simulink model "model"  (Simulink 7.8)
settings: Solver=ode45  StartTime=0.0  StopTime=40.0  RelTol=1e-3
libraries: simulink x2
settings Model: Creator=nort  LastModifiedBy=nort

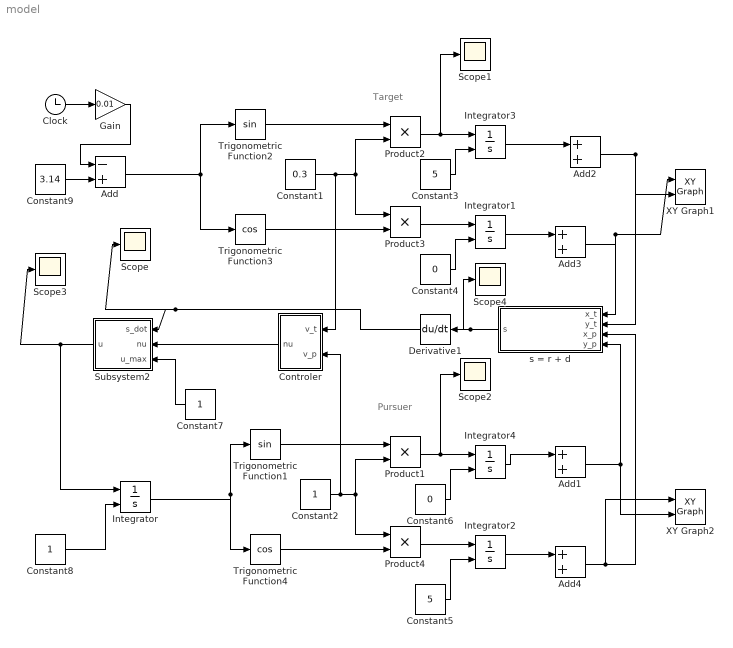
== system model ==
  note: Target
  note: Pursuer
  Add : Sum  Inputs=-+
  Add{1..4} (4 alike) : Sum
  Clock : Clock
  Constant1 : Constant  Value=0.3
  Constant2 : Constant
  Constant3 : Constant  Value=5
  Constant4 : Constant  Value=0
  Constant5 : Constant  Value=5
  Constant6 : Constant  Value=0
  Constant7 : Constant
  Constant8 : Constant
  Constant9 : Constant  Value=3.14
  Controler : Subsystem
  Derivative1 : Derivative
  Gain : Gain  Gain=0.01
  Integrator : Integrator  InitialConditionSource=external  InitialCondition=3.14/4
  Integrator{1..4} (4 alike) : Integrator  InitialConditionSource=external
  Product{1..4} (4 alike) : Product  RndMeth=Zero
  Scope{,1..4} (5 alike) : Scope
      Scope settings: SaveName=ScopeData2
      Scope3 settings: SaveName=ScopeData3
      Scope4 settings: SaveName=ScopeData4
  Subsystem2 : Subsystem
  Trigonometric Function1 : Trigonometry
  Trigonometric Function2 : Trigonometry
  Trigonometric Function3 : Trigonometry  Operator=cos
  Trigonometric Function4 : Trigonometry  Operator=cos
  XY Graph1 : simulink/Sinks/XY Graph  xmin=-15  xmax=15  ymin=-15  ymax=15  st=-1
  XY Graph2 : simulink/Sinks/XY Graph  xmin=-15  xmax=15  ymin=-15  ymax=15  st=-1
  s = r + d : Subsystem
  wires:
  Constant1/1 -> Product2/2, Product3/1, Controler/1(v_t)
  Trigonometric Function2/1 -> Product2/1
  Trigonometric Function3/1 -> Product3/2
  Product2/1 -> Integrator3/1, Scope1/1
  Product3/1 -> Integrator1/1
  Integrator1/1 -> Add3/1
  Add3/1 -> s = r + d/1(x_t), XY Graph1/1
  Add2/1 -> s = r + d/2(y_t), XY Graph1/2
  Integrator3/1 -> Add2/1
  Constant2/1 -> Product1/2, Product4/1, Controler/2(v_p)
  Trigonometric Function1/1 -> Product1/1
  Trigonometric Function4/1 -> Product4/2
  Product1/1 -> Integrator4/1, Scope2/1
  Product4/1 -> Integrator2/1
  Integrator2/1 -> Add4/1
  Add4/1 -> s = r + d/3(x_p), XY Graph2/1
  Add1/1 -> s = r + d/4(y_p), XY Graph2/2
  Integrator4/1 -> Add1/1
  Integrator/1 -> Trigonometric Function1/1, Trigonometric Function4/1
  Constant4/1 -> Integrator1/2
  Constant3/1 -> Integrator3/2
  Constant6/1 -> Integrator4/2
  Constant5/1 -> Integrator2/2
  s = r + d/1(s) -> Derivative1/1, Scope4/1
  Controler/1(nu) -> Subsystem2/2(nu)
  Derivative1/1 -> Subsystem2/1(s_dot), Scope/1
  Constant7/1 -> Subsystem2/3(u_max)
  Subsystem2/1(u) -> Integrator/1, Scope3/1
  Constant8/1 -> Integrator/2
  Add/1 -> Trigonometric Function2/1, Trigonometric Function3/1
  Clock/1 -> Gain/1
  Gain/1 -> Add/1
  Constant9/1 -> Add/2

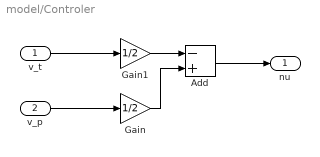
== system model/Controler ==
  v_t : Inport
  v_p : Inport  Port=2
  Add : Sum  Inputs=-+
  Gain : Gain  Gain=1/2
  Gain1 : Gain  Gain=1/2
  nu : Outport
  wires:
  Add/1 -> nu/1
  v_p/1 -> Gain/1
  Gain/1 -> Add/2
  v_t/1 -> Gain1/1
  Gain1/1 -> Add/1

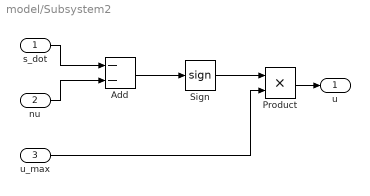
== system model/Subsystem2 ==
  s_dot : Inport
  nu : Inport  Port=2
  u_max : Inport  Port=3
  Add : Sum  Inputs=--
  Product : Product  RndMeth=Zero
  Sign : Signum  ZeroCross=off
  u : Outport
  wires:
  s_dot/1 -> Add/1
  nu/1 -> Add/2
  Add/1 -> Sign/1
  Sign/1 -> Product/1
  u_max/1 -> Product/2
  Product/1 -> u/1

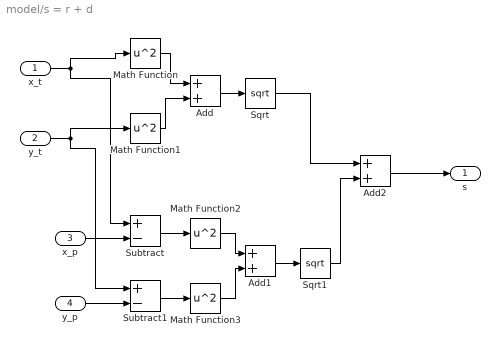
== system model/s = r + d ==
  x_t : Inport
  y_t : Inport  Port=2
  x_p : Inport  Port=3
  y_p : Inport  Port=4
  Add : Sum
  Add1 : Sum
  Add2 : Sum
  Math Function{,1..3} (4 alike) : Math  Operator=square  SaturateOnIntegerOverflow=on
  Sqrt : Sqrt  SaturateOnIntegerOverflow=on
  Sqrt1 : Sqrt  SaturateOnIntegerOverflow=on
  Subtract : Sum  Inputs=+-
  Subtract1 : Sum  Inputs=+-
  s : Outport
  wires:
  Math Function/1 -> Add/1
  Add/1 -> Sqrt/1
  x_t/1 -> Subtract/1, Math Function/1
  y_t/1 -> Subtract1/1, Math Function1/1
  x_p/1 -> Subtract/2
  y_p/1 -> Subtract1/2
  Subtract/1 -> Math Function2/1
  Math Function1/1 -> Add/2
  Subtract1/1 -> Math Function3/1
  Math Function2/1 -> Add1/1
  Math Function3/1 -> Add1/2
  Add1/1 -> Sqrt1/1
  Sqrt/1 -> Add2/1
  Sqrt1/1 -> Add2/2
  Add2/1 -> s/1
